simulink model "brucy"  (R2024b)
settings: Solver=ode1  StartTime=0.0  StopTime=40  FixedStep=0.001  RelTol=1e-3
InitFcn:
  | para
values from neighbouring files (symbols this model uses):
  g_vector = [0.0; 0.0; 9.81]    [para.m]
  K = eye(3) * 50.0    [para.m]
  Lambda = eye(3) * 40.0    [para.m]
  lambda_a = 0.01    [para.m]
  m = 1    [para.m]
  phi = [0.1 0.2 -0.3 1.0 ... (first row only)    [para.m]
  Q = eye(a_hat_shape_0) * 0.1    [para.m]
  R_inv = inv(R)    [para.m]
libraries: simulink x2
settings Model: Creator=Administrator  LastModifiedBy=Administrator

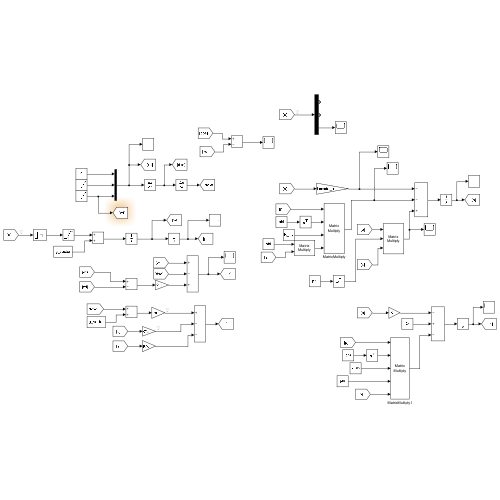
[thumbnail: Simulink's stored preview of the top-level diagram]
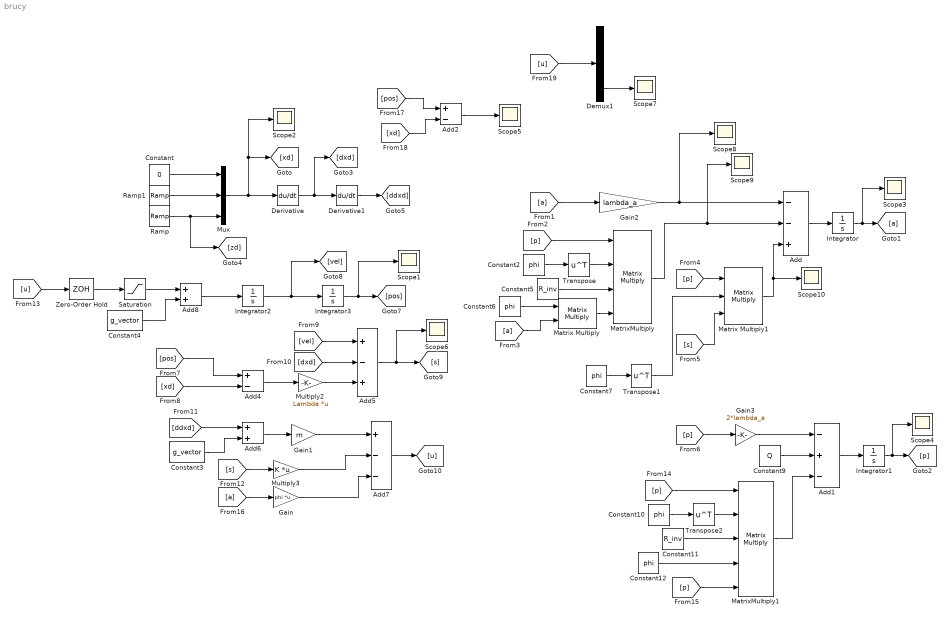
== system brucy ==
  Add : Sum  Inputs=--+
  Add1 : Sum  Inputs=-+-
  Add2 : Sum  Inputs=+-
  Add4 : Sum  Inputs=+-
  Add5 : Sum  Inputs=+-+
  Add6 : Sum
  Add7 : Sum  Inputs=+--
  Add8 : Sum
  Constant : Constant  Value=0
  Constant{2,6..7,10,12} (5 alike) : Constant  Value=phi
  Constant11 : Constant  Value=R_inv
  Constant3 : Constant  Value=g_vector
  Constant4 : Constant  Value=g_vector
  Constant5 : Constant  Value=R_inv
  Constant9 : Constant  Value=Q
  Demux1 : Demux  Outputs=3
  Derivative : Derivative
  Derivative1 : Derivative
  Gain : Gain  Gain=phi  Multiplication=Matrix(K*u)
  Gain1 : Gain  Gain=m
  Gain2 : Gain  Gain=lambda_a
  Gain3 : Gain  Gain=2*lambda_a
  Integrator{,1..3} (4 alike) : Integrator
  Matrix Multiply : Product  Multiplication=Matrix(*)
  Matrix Multiply1 : Product  Inputs=3  Multiplication=Matrix(*)
  MatrixMultiply : Product  Inputs=4  Multiplication=Matrix(*)
  MatrixMultiply1 : Product  Inputs=5  Multiplication=Matrix(*)
  Multiply2 : Gain  Gain=Lambda  Multiplication=Matrix(K*u)
  Multiply3 : Gain  Gain=K  Multiplication=Matrix(K*u)
  Mux : Mux  Inputs=3
  Ramp : simulink/Sources/Ramp  slope=-2  start=0  InitialOutput=0
  Ramp1 : simulink/Sources/Ramp  slope=0  start=0  InitialOutput=0
  Saturation : Saturate  UpperLimit=0  LowerLimit=-20
  Scope{1..10} (10 alike) : Scope
  Transpose : Math  Operator=transpose
  Transpose1 : Math  Operator=transpose
  Transpose2 : Math  Operator=transpose
  Zero-Order Hold : ZeroOrderHold  SampleTime=0.01
  wires:
  Constant/1 -> Mux/1
  Ramp1/1 -> Mux/2
  Ramp/1 -> [zd], Mux/3
  Mux/1 -> Derivative/1, Scope2/1, [xd]
  Derivative/1 -> Derivative1/1, [dxd]
  Derivative1/1 -> [ddxd]
  Integrator3/1 -> Scope1/1, [pos]
  [vel] -> Add5/1
  Gain1/1 -> Add7/1
  Add6/1 -> Gain1/1
  [s] -> Multiply3/1
  Add4/1 -> Multiply2/1
  Add7/1 -> [u]
  [ddxd] -> Add6/1
  [xd] -> Add4/2
  Constant3/1 -> Add6/2
  Add5/1 -> Scope6/1, [s]
  Multiply3/1 -> Add7/2
  [pos] -> Add4/1
  Integrator2/1 -> [vel], Integrator3/1
  Multiply2/1 -> Add5/3
  [dxd] -> Add5/2
  Constant4/1 -> Add8/2
  Add8/1 -> Integrator2/1
  Gain/1 -> Add7/3
  Integrator/1 -> Scope3/1, [a]
  Add/1 -> Integrator/1
  [a] -> Gain2/1
  Gain2/1 -> Scope8/1, Add/1
  Add1/1 -> Integrator1/1
  Integrator1/1 -> Scope4/1, [p]
  [p] -> MatrixMultiply/1
  Transpose/1 -> MatrixMultiply/2
  Constant2/1 -> Transpose/1
  Constant5/1 -> MatrixMultiply/3
  Matrix Multiply/1 -> MatrixMultiply/4
  Constant6/1 -> Matrix Multiply/1
  [a] -> Matrix Multiply/2
  MatrixMultiply/1 -> Scope9/1, Add/2
  Matrix Multiply1/1 -> Scope10/1, Add/3
  Constant7/1 -> Transpose1/1
  Transpose1/1 -> Matrix Multiply1/2
  [p] -> Matrix Multiply1/1
  [s] -> Matrix Multiply1/3
  Gain3/1 -> Add1/1
  Constant9/1 -> Add1/2
  Constant12/1 -> MatrixMultiply1/4
  Constant11/1 -> MatrixMultiply1/3
  Constant10/1 -> Transpose2/1
  Transpose2/1 -> MatrixMultiply1/2
  [p] -> MatrixMultiply1/1
  MatrixMultiply1/1 -> Add1/3
  [p] -> MatrixMultiply1/5
  [a] -> Gain/1
  [p] -> Gain3/1
  Saturation/1 -> Add8/1
  Zero-Order Hold/1 -> Saturation/1
  [u] -> Zero-Order Hold/1
  Add2/1 -> Scope5/1
  [u] -> Demux1/1
  Demux1/3 -> Scope7/1
  [pos] -> Add2/1
  [xd] -> Add2/2
